simulink model "Part5"  (R2017b)
settings: Solver=VariableStepAuto  StartTime=0.0  StopTime=100  RelTol=1e-3
settings Model: Creator=Yazdanpanah  LastModifiedBy=admin
settings DataIOCC: ReturnWorkspaceOutputs=on
settings SFSimCC: SimUseLocalCustomCode=on
settings RTWCC: RTWUseLocalCustomCode=on
settings CodeAppCC: StateflowObjectComments=on

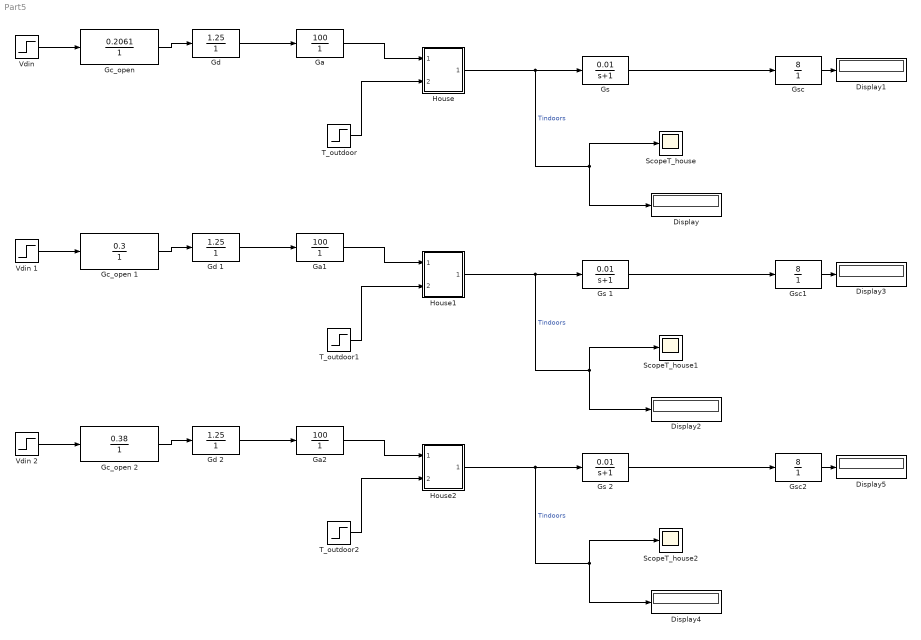
== system Part5 ==
  Display{,1..5} (6 alike) : Display
  Ga : TransferFcn  Numerator=[100]  Denominator=[1 ]
  Ga1 : TransferFcn  Numerator=[100]  Denominator=[1 ]
  Ga2 : TransferFcn  Numerator=[100]  Denominator=[1 ]
  "Gc_open " : TransferFcn  Numerator=[0.2061]  Denominator=[1 ]
  Gc_open 1 : TransferFcn  Numerator=[0.3]  Denominator=[1 ]
  Gc_open 2 : TransferFcn  Numerator=[0.38]  Denominator=[1 ]
  "Gd " : TransferFcn  Numerator=[1.25]  Denominator=[1 ]
  Gd 1 : TransferFcn  Numerator=[1.25]  Denominator=[1 ]
  Gd 2 : TransferFcn  Numerator=[1.25]  Denominator=[1 ]
  "Gs " : TransferFcn  Numerator=[0.01]  Denominator=[1 1]
  Gs 1 : TransferFcn  Numerator=[0.01]  Denominator=[1 1]
  Gs 2 : TransferFcn  Numerator=[0.01]  Denominator=[1 1]
  Gsc : TransferFcn  Numerator=[8]  Denominator=[1 ]
  Gsc1 : TransferFcn  Numerator=[8]  Denominator=[1 ]
  Gsc2 : TransferFcn  Numerator=[8]  Denominator=[1 ]
  House : Subsystem
      mask Display: image(fullfile(matlabroot,'toolbox','simulink','simdemos','simgeneral','images','HouseHeatHousePix.svg'))
  House1 : Subsystem
      mask Display: image(fullfile(matlabroot,'toolbox','simulink','simdemos','simgeneral','images','HouseHeatHousePix.svg'))
  House2 : Subsystem
      mask Display: image(fullfile(matlabroot,'toolbox','simulink','simdemos','simgeneral','images','HouseHeatHousePix.svg'))
  ScopeT_house : Scope
  ScopeT_house1 : Scope
  ScopeT_house2 : Scope
  T_outdoor : Step  Time=0  After=15  SampleTime=0
  T_outdoor1 : Step  Time=0  After=15  SampleTime=0
  T_outdoor2 : Step  Time=0  After=15  SampleTime=0
  "Vdin " : Step  Time=0  After=10  SampleTime=0
  Vdin 1 : Step  Time=0  After=10  SampleTime=0
  Vdin 2 : Step  Time=0  After=10  SampleTime=0
  wires:
  "Gd "/1 -> Ga/1
  T_outdoor/1 -> House/2(Outdoor Temp Tout)
  House/1(Room Temp Troom) -> Display/1, ScopeT_house/1, "Gs "/1  "Tindoors"
  "Gs "/1 -> Gsc/1
  Ga/1 -> House/1(Heater QDot In)
  "Vdin "/1 -> "Gc_open "/1
  "Gc_open "/1 -> "Gd "/1
  Gsc/1 -> Display1/1
  Gd 1/1 -> Ga1/1
  Gc_open 1/1 -> Gd 1/1
  Gsc1/1 -> Display3/1
  T_outdoor1/1 -> House1/2(Outdoor Temp Tout)
  Vdin 1/1 -> Gc_open 1/1
  House1/1(Room Temp Troom) -> Display2/1, ScopeT_house1/1, Gs 1/1  "Tindoors"
  Gs 1/1 -> Gsc1/1
  Ga1/1 -> House1/1(Heater QDot In)
  Gd 2/1 -> Ga2/1
  Gc_open 2/1 -> Gd 2/1
  Gsc2/1 -> Display5/1
  T_outdoor2/1 -> House2/2(Outdoor Temp Tout)
  Vdin 2/1 -> Gc_open 2/1
  House2/1(Room Temp Troom) -> Display4/1, ScopeT_house2/1, Gs 2/1  "Tindoors"
  Gs 2/1 -> Gsc2/1
  Ga2/1 -> House2/1(Heater QDot In)

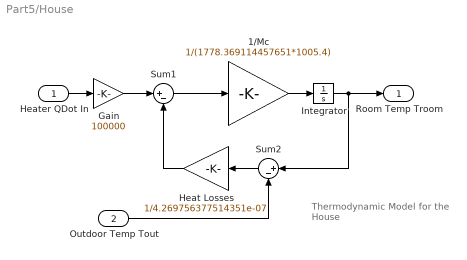
== system Part5/House ==
  note: Thermodynamic Model
      | for the House
  Heater QDot In : Inport
  Outdoor Temp Tout : Inport  Port=2
  1/Mc : Gain  Gain=1/(1778.369114457651*1005.4)  SaturateOnIntegerOverflow=on  OutDataTypeStr=Inherit: Same as input  ParamDataTypeStr=Inherit: Same as input
  Gain : Gain  Gain=100000
  Heat Losses : Gain  Gain=1/4.269756377514351e-07  SaturateOnIntegerOverflow=on  OutDataTypeStr=Inherit: Same as input  ParamDataTypeStr=Inherit: Same as input
  Integrator : Integrator  InitialCondition=20
  Sum1 : Sum  Inputs=|+-  SaturateOnIntegerOverflow=on  InputSameDT=on  OutDataTypeStr=Inherit: Same as first input
  Sum2 : Sum  Inputs=|+-  SaturateOnIntegerOverflow=on  InputSameDT=on  OutDataTypeStr=Inherit: Same as first input
  Room Temp Troom : Outport  InitialOutput=0
  wires:
  Outdoor Temp Tout/1 -> Sum2/2
  Heater QDot In/1 -> Gain/1
  Sum1/1 -> 1/Mc/1
  Sum2/1 -> Heat Losses/1
  Heat Losses/1 -> Sum1/2
  1/Mc/1 -> Integrator/1
  Integrator/1 -> Sum2/1, Room Temp Troom/1
  Gain/1 -> Sum1/1

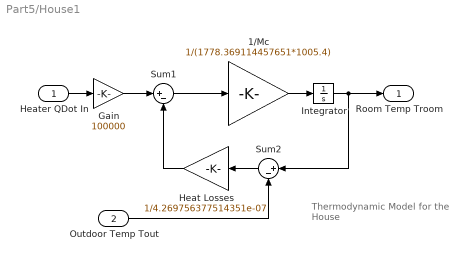
== system Part5/House1 ==
  note: Thermodynamic Model
      | for the House
  Heater QDot In : Inport
  Outdoor Temp Tout : Inport  Port=2
  1/Mc : Gain  Gain=1/(1778.369114457651*1005.4)  SaturateOnIntegerOverflow=on  OutDataTypeStr=Inherit: Same as input  ParamDataTypeStr=Inherit: Same as input
  Gain : Gain  Gain=100000
  Heat Losses : Gain  Gain=1/4.269756377514351e-07  SaturateOnIntegerOverflow=on  OutDataTypeStr=Inherit: Same as input  ParamDataTypeStr=Inherit: Same as input
  Integrator : Integrator  InitialCondition=20
  Sum1 : Sum  Inputs=|+-  SaturateOnIntegerOverflow=on  InputSameDT=on  OutDataTypeStr=Inherit: Same as first input
  Sum2 : Sum  Inputs=|+-  SaturateOnIntegerOverflow=on  InputSameDT=on  OutDataTypeStr=Inherit: Same as first input
  Room Temp Troom : Outport  InitialOutput=0
  wires:
  Outdoor Temp Tout/1 -> Sum2/2
  Heater QDot In/1 -> Gain/1
  Sum1/1 -> 1/Mc/1
  Sum2/1 -> Heat Losses/1
  Heat Losses/1 -> Sum1/2
  1/Mc/1 -> Integrator/1
  Integrator/1 -> Sum2/1, Room Temp Troom/1
  Gain/1 -> Sum1/1

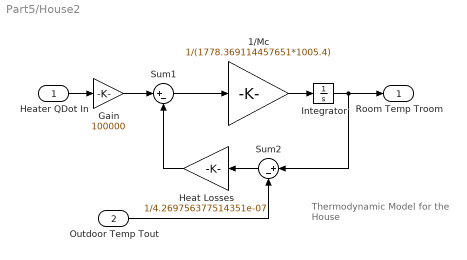
== system Part5/House2 ==
  note: Thermodynamic Model
      | for the House
  Heater QDot In : Inport
  Outdoor Temp Tout : Inport  Port=2
  1/Mc : Gain  Gain=1/(1778.369114457651*1005.4)  SaturateOnIntegerOverflow=on  OutDataTypeStr=Inherit: Same as input  ParamDataTypeStr=Inherit: Same as input
  Gain : Gain  Gain=100000
  Heat Losses : Gain  Gain=1/4.269756377514351e-07  SaturateOnIntegerOverflow=on  OutDataTypeStr=Inherit: Same as input  ParamDataTypeStr=Inherit: Same as input
  Integrator : Integrator  InitialCondition=20
  Sum1 : Sum  Inputs=|+-  SaturateOnIntegerOverflow=on  InputSameDT=on  OutDataTypeStr=Inherit: Same as first input
  Sum2 : Sum  Inputs=|+-  SaturateOnIntegerOverflow=on  InputSameDT=on  OutDataTypeStr=Inherit: Same as first input
  Room Temp Troom : Outport  InitialOutput=0
  wires:
  Outdoor Temp Tout/1 -> Sum2/2
  Heater QDot In/1 -> Gain/1
  Sum1/1 -> 1/Mc/1
  Sum2/1 -> Heat Losses/1
  Heat Losses/1 -> Sum1/2
  1/Mc/1 -> Integrator/1
  Integrator/1 -> Sum2/1, Room Temp Troom/1
  Gain/1 -> Sum1/1
